simulink model "Gearbox_01"  (Simulink 7.9)
settings: Solver=ode45  StartTime=0.0  StopTime=10.0  RelTol=1e-3
undefined symbols (not defined in the file or in its folder): c_getr, d_getr, eta_getr, i_getr, J_last, M_last, Omega_in, T_puls_end, T_puls_start
settings Model: Creator=dep02378  LastModifiedBy=DEP02378

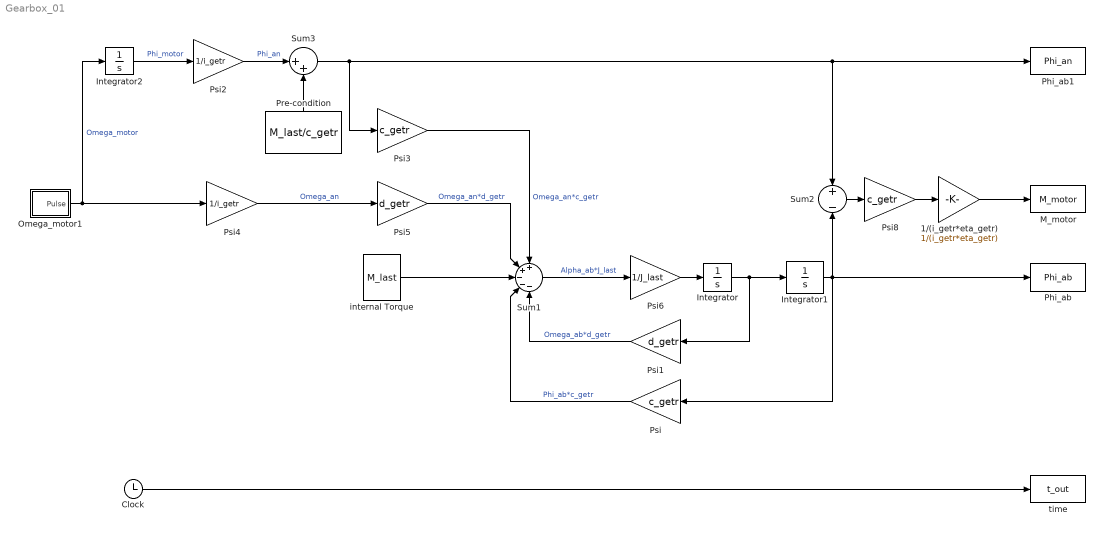
== system Gearbox_01 ==
  1/(i_getr*eta_getr) : Gain  Gain=1/(i_getr*eta_getr)
  Clock : Clock
  Integrator : Integrator
  Integrator1 : Integrator
  Integrator2 : Integrator
  M_motor : ToWorkspace  VariableName=M_motor  SampleTime=-1
  Omega_motor1 : Subsystem
  Phi_ab : ToWorkspace  VariableName=Phi_ab  SampleTime=-1
  Phi_ab1 : ToWorkspace  VariableName=Phi_an  SampleTime=-1
  Pre-condition : Constant  Value=M_last/c_getr
  Psi : Gain  Gain=c_getr
  Psi1 : Gain  Gain=d_getr
  Psi2 : Gain  Gain=1/i_getr
  Psi3 : Gain  Gain=c_getr
  Psi4 : Gain  Gain=1/i_getr
  Psi5 : Gain  Gain=d_getr
  Psi6 : Gain  Gain=1/J_last
  Psi8 : Gain  Gain=c_getr
  Sum1 : Sum  Inputs=++---
  Sum2 : Sum  Inputs=+-
  Sum3 : Sum  Inputs=|++
  internal Torque : Constant  Value=M_last
  time : ToWorkspace  VariableName=t_out  SampleTime=-1
  wires:
  Omega_motor1/1(Pulse) -> Integrator2/1, Psi4/1  "Omega_motor"
  Integrator2/1 -> Psi2/1  "Phi_motor"
  Sum2/1 -> Psi8/1
  1/(i_getr*eta_getr)/1 -> M_motor/1
  Clock/1 -> time/1
  Psi3/1 -> Sum1/1  "Omega_an*c_getr"
  Psi4/1 -> Psi5/1  "Omega_an"
  Psi6/1 -> Integrator/1
  Integrator/1 -> Integrator1/1, Psi1/1
  Sum1/1 -> Psi6/1  "Alpha_ab*J_last"
  Integrator1/1 -> Psi/1, Phi_ab/1, Sum2/2
  Psi1/1 -> Sum1/5  "Omega_ab*d_getr"
  Psi/1 -> Sum1/4  "Phi_ab*c_getr"
  internal Torque/1 -> Sum1/3
  Psi5/1 -> Sum1/2  "Omega_an*d_getr"
  Psi8/1 -> 1/(i_getr*eta_getr)/1
  Sum3/1 -> Psi3/1, Phi_ab1/1, Sum2/1
  Psi2/1 -> Sum3/1  "Phi_an"
  Pre-condition/1 -> Sum3/2

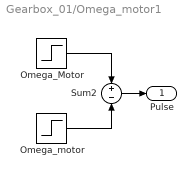
== system Gearbox_01/Omega_motor1 ==
  Omega_Motor : Step  Time=T_puls_start  After=Omega_in  SampleTime=0
  Omega_motor : Step  Time=T_puls_end  After=Omega_in  SampleTime=0
  Sum2 : Sum  Inputs=+-
  Pulse : Outport
  wires:
  Omega_motor/1 -> Sum2/2
  Omega_Motor/1 -> Sum2/1
  Sum2/1 -> Pulse/1
